simulink model "controlled_van_der_pol"  (R2019a)
settings: Solver=VariableStepAuto  StartTime=0.0  StopTime=20  RelTol=1e-3
values from neighbouring files (symbols this model uses):
  mu = vdpParams(3)    [vanDerPolWithFailure.m]    (also in vdp_accommodation_test.m = 0.95; vdp_detection_test.m = 0.95)
  sigma = approximatorParams(end)    [vanDerPolWithFailure.m]    (also in vdp_accommodation_test.m = 0.6; vdp_detection_test.m = 0.6)
  w = 0.9    [vdp_accommodation_test.m]    (also in vdp_detection_test.m)
  y0 = [x0;xHat0; theta0]    [vdp_accommodation_test.m]    (also in vdp_detection_test.m)
settings Model: Creator=fvall  LastModifiedBy=fvall

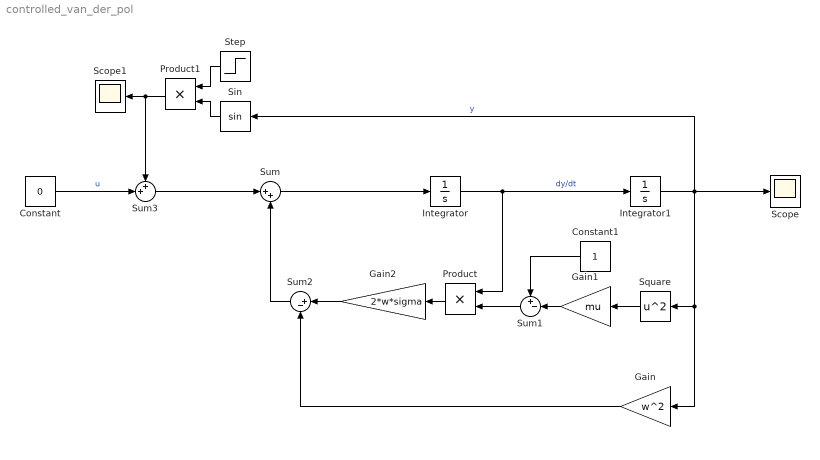
== system controlled_van_der_pol ==
  Constant : Constant  Value=0
  Constant1 : Constant
  Gain : Gain  Gain=w^2
  Gain1 : Gain  Gain=mu
  Gain2 : Gain  Gain=2*w*sigma
  Integrator : Integrator  InitialCondition=y0(2)
  Integrator1 : Integrator  InitialCondition=y0(1)
  Product : Product
  Product1 : Product
  Scope : Scope
  Scope1 : Scope
  Sin : Trigonometry
  Square : Math  Operator=square  SaturateOnIntegerOverflow=on
  Step : Step  Time=10  SampleTime=0
  Sum : Sum  Inputs=|++
  Sum1 : Sum  Inputs=+-|
  Sum2 : Sum  Inputs=|+-
  Sum3 : Sum  Inputs=++|
  wires:
  Sum/1 -> Integrator/1
  Integrator/1 -> Product/1, Integrator1/1  "dy/dt"
  Integrator1/1 -> Sin/1, Scope/1, Gain/1, Square/1  "y"
  Constant1/1 -> Sum1/1
  Gain1/1 -> Sum1/2
  Sum1/1 -> Product/2
  Product/1 -> Gain2/1
  Gain2/1 -> Sum2/1
  Gain/1 -> Sum2/2
  Sum2/1 -> Sum/2
  Square/1 -> Gain1/1
  Constant/1 -> Sum3/2  "u"
  Sum3/1 -> Sum/1
  Sin/1 -> Product1/2
  Step/1 -> Product1/1
  Product1/1 -> Scope1/1, Sum3/1
